simulink model "LAB1__1_2"  (R2020a)
settings: Solver=VariableStepAuto  StartTime=0.0  StopTime=10.0  RelTol=1e-3
settings Model: Creator=Пользователь  LastModifiedBy=Пользователь

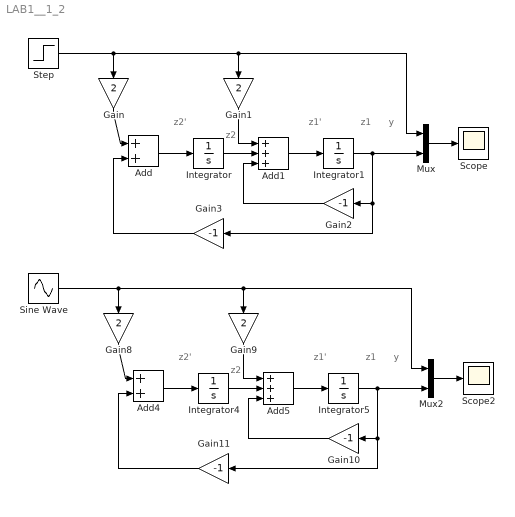
== system LAB1__1_2 ==
  note: z1'
  note: z1
  note: y
  note: z2
  note: z2'
  note: z2'
  note: y
  note: z1
  note: z1'
  note: z2
  Add : Sum
  Add1 : Sum  Inputs=+++
  Add4 : Sum
  Add5 : Sum  Inputs=+++
  Gain{,1,8..9} (4 alike) : Gain  Gain=2
  Gain{2..3,10..11} (4 alike) : Gain  Gain=-1
  Integrator{,1,4..5} (4 alike) : Integrator
  Mux : Mux  Inputs=2
  Mux2 : Mux  Inputs=2
  Scope : Scope
  Scope2 : Scope
  Sine Wave : Sin  Amplitude=2  SampleTime=0
  Step : Step  Time=0.5  SampleTime=0
  wires:
  Step/1 -> Gain/1, Mux/1, Gain1/1
  Gain/1 -> Add/1
  Add/1 -> Integrator/1
  Integrator/1 -> Add1/2
  Gain1/1 -> Add1/1
  Add1/1 -> Integrator1/1
  Integrator1/1 -> Mux/2, Gain3/1, Gain2/1
  Gain2/1 -> Add1/3
  Gain3/1 -> Add/2
  Mux/1 -> Scope/1
  Mux2/1 -> Scope2/1
  Add5/1 -> Integrator5/1
  Gain9/1 -> Add5/1
  Gain10/1 -> Add5/3
  Gain11/1 -> Add4/2
  Gain8/1 -> Add4/1
  Add4/1 -> Integrator4/1
  Integrator4/1 -> Add5/2
  Sine Wave/1 -> Gain8/1, Mux2/1, Gain9/1
  Integrator5/1 -> Mux2/2, Gain11/1, Gain10/1
